simulink model "elevator"  (R2020a)
settings: Solver=VariableStepAuto  StartTime=0.0  StopTime=inf  RelTol=1e-3
PreLoadFcn:
  | slplc.api.loadDataTypes;
undefined symbols (not defined in the file): BOOL, DINT, INT, slplc
libraries: simulink x1
(part 34 of 38)

== matlab function elevator/PLCControllerSuite/__Logic/Task/Program/__Logic/OTE28/__Format ==
  data: BlockEnable input; RungIn input; RungOut input; data input
function setBlockFormat(BlockEnable, RungIn, RungOut, data)

if data~=0 && data~=1
    error('slplc:inivalidBooleanValue', 'Invalid boolean value %d', data);
end
data = logical(data);

% set parent block colors
coder.extrinsic('slplc.utils.setBlockAppearance');
persistent lastBlockEnable lastRungIn lastRungOut lastData isInit lastAnimation lastDataShow;
if isempty(lastBlockEnable)
    lastBlockEnable = true;
end
if isempty(lastRungIn)
    lastRungIn = false;
end
if isempty(lastRungOut)
    lastRungOut = false;
end
if isempty(lastData)
    lastData = data;
end
if isempty(isInit)
    isInit = true;
else
    isInit = false;
end
if isempty(lastAnimation)
    lastAnimation = false;
end
if isempty(lastDataShow)
    lastDataShow = false;
end

[animation, dataShow] = slplc.utils.setBlockAppearance('set', '%<PLCOperandTag>', {}, {}, ...
    ' = ', {'ForegroundColor'}, ...
    isInit,  ...
    BlockEnable, lastBlockEnable, ...
    RungIn,  lastRungIn, ...
    RungOut, lastRungOut, ...
    data, lastData, ...
    lastAnimation, lastDataShow);

lastBlockEnable = BlockEnable;
lastRungIn      = RungIn;
lastRungOut     = RungOut;
lastData        = data;
lastAnimation   = animation;
lastDataShow    = dataShow;
end

== matlab function elevator/PLCControllerSuite/__Logic/Task/Program/__Logic/XIC72/__Format ==
  data: BlockEnable input; RungIn input; RungOut input; data input
function setBlockFormat(BlockEnable, RungIn, RungOut, data)

if data~=0 && data~=1
    error('slplc:inivalidBooleanValue', 'Invalid boolean value %d', data);
end
data = logical(data);

% set parent block colors
coder.extrinsic('slplc.utils.setBlockAppearance');
persistent lastBlockEnable lastRungIn lastRungOut lastData isInit lastAnimation lastDataShow;
if isempty(lastBlockEnable)
    lastBlockEnable = true;
end
if isempty(lastRungIn)
    lastRungIn = false;
end
if isempty(lastRungOut)
    lastRungOut = false;
end
if isempty(lastData)
    lastData = data;
end
if isempty(isInit)
    isInit = true;
else
    isInit = false;
end
if isempty(lastAnimation)
    lastAnimation = false;
end
if isempty(lastDataShow)
    lastDataShow = false;
end

[animation, dataShow] = slplc.utils.setBlockAppearance('set', '%<PLCOperandTag>', {}, {}, ...
    ' = ', {'ForegroundColor'}, ...
    isInit,  ...
    BlockEnable, lastBlockEnable, ...
    RungIn,  lastRungIn, ...
    RungOut, lastRungOut, ...
    data, lastData, ...
    lastAnimation, lastDataShow);

lastBlockEnable = BlockEnable;
lastRungIn      = RungIn;
lastRungOut     = RungOut;
lastData        = data;
lastAnimation   = animation;
lastDataShow    = dataShow;
end

== matlab function elevator/PLCControllerSuite/__Logic/Task/Program/__Logic/XIO29/__Format ==
  data: BlockEnable input; RungIn input; RungOut input; data input
function setBlockFormat(BlockEnable, RungIn, RungOut, data)

if data~=0 && data~=1
    error('slplc:inivalidBooleanValue', 'Invalid boolean value %d', data);
end
data = logical(data);

% set parent block colors
coder.extrinsic('slplc.utils.setBlockAppearance');
persistent lastBlockEnable lastRungIn lastRungOut lastData isInit lastAnimation lastDataShow;
if isempty(lastBlockEnable)
    lastBlockEnable = true;
end
if isempty(lastRungIn)
    lastRungIn = false;
end
if isempty(lastRungOut)
    lastRungOut = false;
end
if isempty(lastData)
    lastData = data;
end
if isempty(isInit)
    isInit = true;
else
    isInit = false;
end
if isempty(lastAnimation)
    lastAnimation = false;
end
if isempty(lastDataShow)
    lastDataShow = false;
end

[animation, dataShow] = slplc.utils.setBlockAppearance('set', '%<PLCOperandTag>', {}, {}, ...
    ' = ', {'ForegroundColor'}, ...
    isInit,  ...
    BlockEnable, lastBlockEnable, ...
    RungIn,  lastRungIn, ...
    RungOut, lastRungOut, ...
    data, lastData, ...
    lastAnimation, lastDataShow);

lastBlockEnable = BlockEnable;
lastRungIn      = RungIn;
lastRungOut     = RungOut;
lastData        = data;
lastAnimation   = animation;
lastDataShow    = dataShow;
end

== matlab function elevator/PLCControllerSuite/__Logic/Task/Program/__Logic/XIC92/__Format ==
  data: BlockEnable input; RungIn input; RungOut input; data input
function setBlockFormat(BlockEnable, RungIn, RungOut, data)

if data~=0 && data~=1
    error('slplc:inivalidBooleanValue', 'Invalid boolean value %d', data);
end
data = logical(data);

% set parent block colors
coder.extrinsic('slplc.utils.setBlockAppearance');
persistent lastBlockEnable lastRungIn lastRungOut lastData isInit lastAnimation lastDataShow;
if isempty(lastBlockEnable)
    lastBlockEnable = true;
end
if isempty(lastRungIn)
    lastRungIn = false;
end
if isempty(lastRungOut)
    lastRungOut = false;
end
if isempty(lastData)
    lastData = data;
end
if isempty(isInit)
    isInit = true;
else
    isInit = false;
end
if isempty(lastAnimation)
    lastAnimation = false;
end
if isempty(lastDataShow)
    lastDataShow = false;
end

[animation, dataShow] = slplc.utils.setBlockAppearance('set', '%<PLCOperandTag>', {}, {}, ...
    ' = ', {'ForegroundColor'}, ...
    isInit,  ...
    BlockEnable, lastBlockEnable, ...
    RungIn,  lastRungIn, ...
    RungOut, lastRungOut, ...
    data, lastData, ...
    lastAnimation, lastDataShow);

lastBlockEnable = BlockEnable;
lastRungIn      = RungIn;
lastRungOut     = RungOut;
lastData        = data;
lastAnimation   = animation;
lastDataShow    = dataShow;
end

== matlab function elevator/PLCControllerSuite/__Logic/Task/Program/__Logic/Junction3/__Format ==
  data: BlockEnable input; RungOut input
function setBlockFormat(BlockEnable, RungOut)
% set parent block colors
coder.extrinsic('slplc.utils.setBlockAppearance');
persistent lastBlockEnable isInit lastRungOut lastAnimation lastRungOutShow;
if isempty(lastBlockEnable)
    lastBlockEnable = true;
end

if isempty(isInit)
    isInit = true;
else
    isInit = false;
end

if isempty(lastRungOut)
    lastRungOut = RungOut;
end

if isempty(lastAnimation)
    lastAnimation = false;
end

if isempty(lastRungOutShow)
    lastRungOutShow = false;
end

[animation, dataShow] = slplc.utils.setBlockAppearance('set', '', {'black', 'black'}, {}, ...
    '', {'ForegroundColor', 'BackgroundColor'}, ...
    isInit,  ...
    BlockEnable, lastBlockEnable, ...
    RungOut,   lastRungOut, ...
    RungOut,   lastRungOut, ...
    [],    [], ...
    lastAnimation, lastRungOutShow);

lastBlockEnable     = BlockEnable;
lastRungOut         = RungOut;
lastAnimation       = animation;
lastRungOutShow     = dataShow;
end

== matlab function elevator/PLCControllerSuite/__Logic/Task/Program/__Logic/XIC99/__Format ==
  data: BlockEnable input; RungIn input; RungOut input; data input
function setBlockFormat(BlockEnable, RungIn, RungOut, data)

if data~=0 && data~=1
    error('slplc:inivalidBooleanValue', 'Invalid boolean value %d', data);
end
data = logical(data);

% set parent block colors
coder.extrinsic('slplc.utils.setBlockAppearance');
persistent lastBlockEnable lastRungIn lastRungOut lastData isInit lastAnimation lastDataShow;
if isempty(lastBlockEnable)
    lastBlockEnable = true;
end
if isempty(lastRungIn)
    lastRungIn = false;
end
if isempty(lastRungOut)
    lastRungOut = false;
end
if isempty(lastData)
    lastData = data;
end
if isempty(isInit)
    isInit = true;
else
    isInit = false;
end
if isempty(lastAnimation)
    lastAnimation = false;
end
if isempty(lastDataShow)
    lastDataShow = false;
end

[animation, dataShow] = slplc.utils.setBlockAppearance('set', '%<PLCOperandTag>', {}, {}, ...
    ' = ', {'ForegroundColor'}, ...
    isInit,  ...
    BlockEnable, lastBlockEnable, ...
    RungIn,  lastRungIn, ...
    RungOut, lastRungOut, ...
    data, lastData, ...
    lastAnimation, lastDataShow);

lastBlockEnable = BlockEnable;
lastRungIn      = RungIn;
lastRungOut     = RungOut;
lastData        = data;
lastAnimation   = animation;
lastDataShow    = dataShow;
end

== matlab function elevator/PLCControllerSuite/__Logic/Task/Program/__Logic/XIO18/__Format ==
  data: BlockEnable input; RungIn input; RungOut input; data input
function setBlockFormat(BlockEnable, RungIn, RungOut, data)

if data~=0 && data~=1
    error('slplc:inivalidBooleanValue', 'Invalid boolean value %d', data);
end
data = logical(data);

% set parent block colors
coder.extrinsic('slplc.utils.setBlockAppearance');
persistent lastBlockEnable lastRungIn lastRungOut lastData isInit lastAnimation lastDataShow;
if isempty(lastBlockEnable)
    lastBlockEnable = true;
end
if isempty(lastRungIn)
    lastRungIn = false;
end
if isempty(lastRungOut)
    lastRungOut = false;
end
if isempty(lastData)
    lastData = data;
end
if isempty(isInit)
    isInit = true;
else
    isInit = false;
end
if isempty(lastAnimation)
    lastAnimation = false;
end
if isempty(lastDataShow)
    lastDataShow = false;
end

[animation, dataShow] = slplc.utils.setBlockAppearance('set', '%<PLCOperandTag>', {}, {}, ...
    ' = ', {'ForegroundColor'}, ...
    isInit,  ...
    BlockEnable, lastBlockEnable, ...
    RungIn,  lastRungIn, ...
    RungOut, lastRungOut, ...
    data, lastData, ...
    lastAnimation, lastDataShow);

lastBlockEnable = BlockEnable;
lastRungIn      = RungIn;
lastRungOut     = RungOut;
lastData        = data;
lastAnimation   = animation;
lastDataShow    = dataShow;
end

== matlab function elevator/PLCControllerSuite/__Logic/Task/Program/__Logic/XIO19/__Format ==
  data: BlockEnable input; RungIn input; RungOut input; data input
function setBlockFormat(BlockEnable, RungIn, RungOut, data)

if data~=0 && data~=1
    error('slplc:inivalidBooleanValue', 'Invalid boolean value %d', data);
end
data = logical(data);

% set parent block colors
coder.extrinsic('slplc.utils.setBlockAppearance');
persistent lastBlockEnable lastRungIn lastRungOut lastData isInit lastAnimation lastDataShow;
if isempty(lastBlockEnable)
    lastBlockEnable = true;
end
if isempty(lastRungIn)
    lastRungIn = false;
end
if isempty(lastRungOut)
    lastRungOut = false;
end
if isempty(lastData)
    lastData = data;
end
if isempty(isInit)
    isInit = true;
else
    isInit = false;
end
if isempty(lastAnimation)
    lastAnimation = false;
end
if isempty(lastDataShow)
    lastDataShow = false;
end

[animation, dataShow] = slplc.utils.setBlockAppearance('set', '%<PLCOperandTag>', {}, {}, ...
    ' = ', {'ForegroundColor'}, ...
    isInit,  ...
    BlockEnable, lastBlockEnable, ...
    RungIn,  lastRungIn, ...
    RungOut, lastRungOut, ...
    data, lastData, ...
    lastAnimation, lastDataShow);

lastBlockEnable = BlockEnable;
lastRungIn      = RungIn;
lastRungOut     = RungOut;
lastData        = data;
lastAnimation   = animation;
lastDataShow    = dataShow;
end

== matlab function elevator/PLCControllerSuite/__Logic/Task/Program/__Logic/XIO20/__Format ==
  data: BlockEnable input; RungIn input; RungOut input; data input
function setBlockFormat(BlockEnable, RungIn, RungOut, data)

if data~=0 && data~=1
    error('slplc:inivalidBooleanValue', 'Invalid boolean value %d', data);
end
data = logical(data);

% set parent block colors
coder.extrinsic('slplc.utils.setBlockAppearance');
persistent lastBlockEnable lastRungIn lastRungOut lastData isInit lastAnimation lastDataShow;
if isempty(lastBlockEnable)
    lastBlockEnable = true;
end
if isempty(lastRungIn)
    lastRungIn = false;
end
if isempty(lastRungOut)
    lastRungOut = false;
end
if isempty(lastData)
    lastData = data;
end
if isempty(isInit)
    isInit = true;
else
    isInit = false;
end
if isempty(lastAnimation)
    lastAnimation = false;
end
if isempty(lastDataShow)
    lastDataShow = false;
end

[animation, dataShow] = slplc.utils.setBlockAppearance('set', '%<PLCOperandTag>', {}, {}, ...
    ' = ', {'ForegroundColor'}, ...
    isInit,  ...
    BlockEnable, lastBlockEnable, ...
    RungIn,  lastRungIn, ...
    RungOut, lastRungOut, ...
    data, lastData, ...
    lastAnimation, lastDataShow);

lastBlockEnable = BlockEnable;
lastRungIn      = RungIn;
lastRungOut     = RungOut;
lastData        = data;
lastAnimation   = animation;
lastDataShow    = dataShow;
end

== matlab function elevator/PLCControllerSuite/__Logic/Task/Program/__Logic/XIO21/__Format ==
  data: BlockEnable input; RungIn input; RungOut input; data input
function setBlockFormat(BlockEnable, RungIn, RungOut, data)

if data~=0 && data~=1
    error('slplc:inivalidBooleanValue', 'Invalid boolean value %d', data);
end
data = logical(data);

% set parent block colors
coder.extrinsic('slplc.utils.setBlockAppearance');
persistent lastBlockEnable lastRungIn lastRungOut lastData isInit lastAnimation lastDataShow;
if isempty(lastBlockEnable)
    lastBlockEnable = true;
end
if isempty(lastRungIn)
    lastRungIn = false;
end
if isempty(lastRungOut)
    lastRungOut = false;
end
if isempty(lastData)
    lastData = data;
end
if isempty(isInit)
    isInit = true;
else
    isInit = false;
end
if isempty(lastAnimation)
    lastAnimation = false;
end
if isempty(lastDataShow)
    lastDataShow = false;
end

[animation, dataShow] = slplc.utils.setBlockAppearance('set', '%<PLCOperandTag>', {}, {}, ...
    ' = ', {'ForegroundColor'}, ...
    isInit,  ...
    BlockEnable, lastBlockEnable, ...
    RungIn,  lastRungIn, ...
    RungOut, lastRungOut, ...
    data, lastData, ...
    lastAnimation, lastDataShow);

lastBlockEnable = BlockEnable;
lastRungIn      = RungIn;
lastRungOut     = RungOut;
lastData        = data;
lastAnimation   = animation;
lastDataShow    = dataShow;
end

== matlab function elevator/PLCControllerSuite/__Logic/Task/Program/__Logic/XIO22/__Format ==
  data: BlockEnable input; RungIn input; RungOut input; data input
function setBlockFormat(BlockEnable, RungIn, RungOut, data)

if data~=0 && data~=1
    error('slplc:inivalidBooleanValue', 'Invalid boolean value %d', data);
end
data = logical(data);

% set parent block colors
coder.extrinsic('slplc.utils.setBlockAppearance');
persistent lastBlockEnable lastRungIn lastRungOut lastData isInit lastAnimation lastDataShow;
if isempty(lastBlockEnable)
    lastBlockEnable = true;
end
if isempty(lastRungIn)
    lastRungIn = false;
end
if isempty(lastRungOut)
    lastRungOut = false;
end
if isempty(lastData)
    lastData = data;
end
if isempty(isInit)
    isInit = true;
else
    isInit = false;
end
if isempty(lastAnimation)
    lastAnimation = false;
end
if isempty(lastDataShow)
    lastDataShow = false;
end

[animation, dataShow] = slplc.utils.setBlockAppearance('set', '%<PLCOperandTag>', {}, {}, ...
    ' = ', {'ForegroundColor'}, ...
    isInit,  ...
    BlockEnable, lastBlockEnable, ...
    RungIn,  lastRungIn, ...
    RungOut, lastRungOut, ...
    data, lastData, ...
    lastAnimation, lastDataShow);

lastBlockEnable = BlockEnable;
lastRungIn      = RungIn;
lastRungOut     = RungOut;
lastData        = data;
lastAnimation   = animation;
lastDataShow    = dataShow;
end

== matlab function elevator/PLCControllerSuite/__Logic/Task/Program/__Logic/XIO34/__Format ==
  data: BlockEnable input; RungIn input; RungOut input; data input
function setBlockFormat(BlockEnable, RungIn, RungOut, data)

if data~=0 && data~=1
    error('slplc:inivalidBooleanValue', 'Invalid boolean value %d', data);
end
data = logical(data);

% set parent block colors
coder.extrinsic('slplc.utils.setBlockAppearance');
persistent lastBlockEnable lastRungIn lastRungOut lastData isInit lastAnimation lastDataShow;
if isempty(lastBlockEnable)
    lastBlockEnable = true;
end
if isempty(lastRungIn)
    lastRungIn = false;
end
if isempty(lastRungOut)
    lastRungOut = false;
end
if isempty(lastData)
    lastData = data;
end
if isempty(isInit)
    isInit = true;
else
    isInit = false;
end
if isempty(lastAnimation)
    lastAnimation = false;
end
if isempty(lastDataShow)
    lastDataShow = false;
end

[animation, dataShow] = slplc.utils.setBlockAppearance('set', '%<PLCOperandTag>', {}, {}, ...
    ' = ', {'ForegroundColor'}, ...
    isInit,  ...
    BlockEnable, lastBlockEnable, ...
    RungIn,  lastRungIn, ...
    RungOut, lastRungOut, ...
    data, lastData, ...
    lastAnimation, lastDataShow);

lastBlockEnable = BlockEnable;
lastRungIn      = RungIn;
lastRungOut     = RungOut;
lastData        = data;
lastAnimation   = animation;
lastDataShow    = dataShow;
end

== matlab function elevator/PLCControllerSuite/__Logic/Task/Program/__Logic/Junction28/__Format ==
  data: BlockEnable input; RungOut input
function setBlockFormat(BlockEnable, RungOut)
% set parent block colors
coder.extrinsic('slplc.utils.setBlockAppearance');
persistent lastBlockEnable isInit lastRungOut lastAnimation lastRungOutShow;
if isempty(lastBlockEnable)
    lastBlockEnable = true;
end

if isempty(isInit)
    isInit = true;
else
    isInit = false;
end

if isempty(lastRungOut)
    lastRungOut = RungOut;
end

if isempty(lastAnimation)
    lastAnimation = false;
end

if isempty(lastRungOutShow)
    lastRungOutShow = false;
end

[animation, dataShow] = slplc.utils.setBlockAppearance('set', '', {'black', 'black'}, {}, ...
    '', {'ForegroundColor', 'BackgroundColor'}, ...
    isInit,  ...
    BlockEnable, lastBlockEnable, ...
    RungOut,   lastRungOut, ...
    RungOut,   lastRungOut, ...
    [],    [], ...
    lastAnimation, lastRungOutShow);

lastBlockEnable     = BlockEnable;
lastRungOut         = RungOut;
lastAnimation       = animation;
lastRungOutShow     = dataShow;
end

== matlab function elevator/PLCControllerSuite/__Logic/Task/Program/__Logic/OTE3/__Format ==
  data: BlockEnable input; RungIn input; RungOut input; data input
function setBlockFormat(BlockEnable, RungIn, RungOut, data)

if data~=0 && data~=1
    error('slplc:inivalidBooleanValue', 'Invalid boolean value %d', data);
end
data = logical(data);

% set parent block colors
coder.extrinsic('slplc.utils.setBlockAppearance');
persistent lastBlockEnable lastRungIn lastRungOut lastData isInit lastAnimation lastDataShow;
if isempty(lastBlockEnable)
    lastBlockEnable = true;
end
if isempty(lastRungIn)
    lastRungIn = false;
end
if isempty(lastRungOut)
    lastRungOut = false;
end
if isempty(lastData)
    lastData = data;
end
if isempty(isInit)
    isInit = true;
else
    isInit = false;
end
if isempty(lastAnimation)
    lastAnimation = false;
end
if isempty(lastDataShow)
    lastDataShow = false;
end

[animation, dataShow] = slplc.utils.setBlockAppearance('set', '%<PLCOperandTag>', {}, {}, ...
    ' = ', {'ForegroundColor'}, ...
    isInit,  ...
    BlockEnable, lastBlockEnable, ...
    RungIn,  lastRungIn, ...
    RungOut, lastRungOut, ...
    data, lastData, ...
    lastAnimation, lastDataShow);

lastBlockEnable = BlockEnable;
lastRungIn      = RungIn;
lastRungOut     = RungOut;
lastData        = data;
lastAnimation   = animation;
lastDataShow    = dataShow;
end

== matlab function elevator/PLCControllerSuite/__Logic/Task/Program/__Logic/OTE16/__Format ==
  data: BlockEnable input; RungIn input; RungOut input; data input
function setBlockFormat(BlockEnable, RungIn, RungOut, data)

if data~=0 && data~=1
    error('slplc:inivalidBooleanValue', 'Invalid boolean value %d', data);
end
data = logical(data);

% set parent block colors
coder.extrinsic('slplc.utils.setBlockAppearance');
persistent lastBlockEnable lastRungIn lastRungOut lastData isInit lastAnimation lastDataShow;
if isempty(lastBlockEnable)
    lastBlockEnable = true;
end
if isempty(lastRungIn)
    lastRungIn = false;
end
if isempty(lastRungOut)
    lastRungOut = false;
end
if isempty(lastData)
    lastData = data;
end
if isempty(isInit)
    isInit = true;
else
    isInit = false;
end
if isempty(lastAnimation)
    lastAnimation = false;
end
if isempty(lastDataShow)
    lastDataShow = false;
end

[animation, dataShow] = slplc.utils.setBlockAppearance('set', '%<PLCOperandTag>', {}, {}, ...
    ' = ', {'ForegroundColor'}, ...
    isInit,  ...
    BlockEnable, lastBlockEnable, ...
    RungIn,  lastRungIn, ...
    RungOut, lastRungOut, ...
    data, lastData, ...
    lastAnimation, lastDataShow);

lastBlockEnable = BlockEnable;
lastRungIn      = RungIn;
lastRungOut     = RungOut;
lastData        = data;
lastAnimation   = animation;
lastDataShow    = dataShow;
end

== matlab function elevator/PLCControllerSuite/__Logic/Task/Program/__Logic/XIC90/__Format ==
  data: BlockEnable input; RungIn input; RungOut input; data input
function setBlockFormat(BlockEnable, RungIn, RungOut, data)

if data~=0 && data~=1
    error('slplc:inivalidBooleanValue', 'Invalid boolean value %d', data);
end
data = logical(data);

% set parent block colors
coder.extrinsic('slplc.utils.setBlockAppearance');
persistent lastBlockEnable lastRungIn lastRungOut lastData isInit lastAnimation lastDataShow;
if isempty(lastBlockEnable)
    lastBlockEnable = true;
end
if isempty(lastRungIn)
    lastRungIn = false;
end
if isempty(lastRungOut)
    lastRungOut = false;
end
if isempty(lastData)
    lastData = data;
end
if isempty(isInit)
    isInit = true;
else
    isInit = false;
end
if isempty(lastAnimation)
    lastAnimation = false;
end
if isempty(lastDataShow)
    lastDataShow = false;
end

[animation, dataShow] = slplc.utils.setBlockAppearance('set', '%<PLCOperandTag>', {}, {}, ...
    ' = ', {'ForegroundColor'}, ...
    isInit,  ...
    BlockEnable, lastBlockEnable, ...
    RungIn,  lastRungIn, ...
    RungOut, lastRungOut, ...
    data, lastData, ...
    lastAnimation, lastDataShow);

lastBlockEnable = BlockEnable;
lastRungIn      = RungIn;
lastRungOut     = RungOut;
lastData        = data;
lastAnimation   = animation;
lastDataShow    = dataShow;
end

== matlab function elevator/PLCControllerSuite/__Logic/Task/Program/__Logic/XIC91/__Format ==
  data: BlockEnable input; RungIn input; RungOut input; data input
function setBlockFormat(BlockEnable, RungIn, RungOut, data)

if data~=0 && data~=1
    error('slplc:inivalidBooleanValue', 'Invalid boolean value %d', data);
end
data = logical(data);

% set parent block colors
coder.extrinsic('slplc.utils.setBlockAppearance');
persistent lastBlockEnable lastRungIn lastRungOut lastData isInit lastAnimation lastDataShow;
if isempty(lastBlockEnable)
    lastBlockEnable = true;
end
if isempty(lastRungIn)
    lastRungIn = false;
end
if isempty(lastRungOut)
    lastRungOut = false;
end
if isempty(lastData)
    lastData = data;
end
if isempty(isInit)
    isInit = true;
else
    isInit = false;
end
if isempty(lastAnimation)
    lastAnimation = false;
end
if isempty(lastDataShow)
    lastDataShow = false;
end

[animation, dataShow] = slplc.utils.setBlockAppearance('set', '%<PLCOperandTag>', {}, {}, ...
    ' = ', {'ForegroundColor'}, ...
    isInit,  ...
    BlockEnable, lastBlockEnable, ...
    RungIn,  lastRungIn, ...
    RungOut, lastRungOut, ...
    data, lastData, ...
    lastAnimation, lastDataShow);

lastBlockEnable = BlockEnable;
lastRungIn      = RungIn;
lastRungOut     = RungOut;
lastData        = data;
lastAnimation   = animation;
lastDataShow    = dataShow;
end

== matlab function elevator/PLCControllerSuite/__Logic/Task/Program/__Logic/Junction32/__Format ==
  data: BlockEnable input; RungOut input
function setBlockFormat(BlockEnable, RungOut)
% set parent block colors
coder.extrinsic('slplc.utils.setBlockAppearance');
persistent lastBlockEnable isInit lastRungOut lastAnimation lastRungOutShow;
if isempty(lastBlockEnable)
    lastBlockEnable = true;
end

if isempty(isInit)
    isInit = true;
else
    isInit = false;
end

if isempty(lastRungOut)
    lastRungOut = RungOut;
end

if isempty(lastAnimation)
    lastAnimation = false;
end

if isempty(lastRungOutShow)
    lastRungOutShow = false;
end

[animation, dataShow] = slplc.utils.setBlockAppearance('set', '', {'black', 'black'}, {}, ...
    '', {'ForegroundColor', 'BackgroundColor'}, ...
    isInit,  ...
    BlockEnable, lastBlockEnable, ...
    RungOut,   lastRungOut, ...
    RungOut,   lastRungOut, ...
    [],    [], ...
    lastAnimation, lastRungOutShow);

lastBlockEnable     = BlockEnable;
lastRungOut         = RungOut;
lastAnimation       = animation;
lastRungOutShow     = dataShow;
end

== matlab function elevator/PLCControllerSuite/__Logic/Task/Program/__Logic/OTE21/__Format ==
  data: BlockEnable input; RungIn input; RungOut input; data input
function setBlockFormat(BlockEnable, RungIn, RungOut, data)

if data~=0 && data~=1
    error('slplc:inivalidBooleanValue', 'Invalid boolean value %d', data);
end
data = logical(data);

% set parent block colors
coder.extrinsic('slplc.utils.setBlockAppearance');
persistent lastBlockEnable lastRungIn lastRungOut lastData isInit lastAnimation lastDataShow;
if isempty(lastBlockEnable)
    lastBlockEnable = true;
end
if isempty(lastRungIn)
    lastRungIn = false;
end
if isempty(lastRungOut)
    lastRungOut = false;
end
if isempty(lastData)
    lastData = data;
end
if isempty(isInit)
    isInit = true;
else
    isInit = false;
end
if isempty(lastAnimation)
    lastAnimation = false;
end
if isempty(lastDataShow)
    lastDataShow = false;
end

[animation, dataShow] = slplc.utils.setBlockAppearance('set', '%<PLCOperandTag>', {}, {}, ...
    ' = ', {'ForegroundColor'}, ...
    isInit,  ...
    BlockEnable, lastBlockEnable, ...
    RungIn,  lastRungIn, ...
    RungOut, lastRungOut, ...
    data, lastData, ...
    lastAnimation, lastDataShow);

lastBlockEnable = BlockEnable;
lastRungIn      = RungIn;
lastRungOut     = RungOut;
lastData        = data;
lastAnimation   = animation;
lastDataShow    = dataShow;
end

== matlab function elevator/PLCControllerSuite/__Logic/Task/Program/__Logic/XIC93/__Format ==
  data: BlockEnable input; RungIn input; RungOut input; data input
function setBlockFormat(BlockEnable, RungIn, RungOut, data)

if data~=0 && data~=1
    error('slplc:inivalidBooleanValue', 'Invalid boolean value %d', data);
end
data = logical(data);

% set parent block colors
coder.extrinsic('slplc.utils.setBlockAppearance');
persistent lastBlockEnable lastRungIn lastRungOut lastData isInit lastAnimation lastDataShow;
if isempty(lastBlockEnable)
    lastBlockEnable = true;
end
if isempty(lastRungIn)
    lastRungIn = false;
end
if isempty(lastRungOut)
    lastRungOut = false;
end
if isempty(lastData)
    lastData = data;
end
if isempty(isInit)
    isInit = true;
else
    isInit = false;
end
if isempty(lastAnimation)
    lastAnimation = false;
end
if isempty(lastDataShow)
    lastDataShow = false;
end

[animation, dataShow] = slplc.utils.setBlockAppearance('set', '%<PLCOperandTag>', {}, {}, ...
    ' = ', {'ForegroundColor'}, ...
    isInit,  ...
    BlockEnable, lastBlockEnable, ...
    RungIn,  lastRungIn, ...
    RungOut, lastRungOut, ...
    data, lastData, ...
    lastAnimation, lastDataShow);

lastBlockEnable = BlockEnable;
lastRungIn      = RungIn;
lastRungOut     = RungOut;
lastData        = data;
lastAnimation   = animation;
lastDataShow    = dataShow;
end

== matlab function elevator/PLCControllerSuite/__Logic/Task/Program/__Logic/XIC94/__Format ==
  data: BlockEnable input; RungIn input; RungOut input; data input
function setBlockFormat(BlockEnable, RungIn, RungOut, data)

if data~=0 && data~=1
    error('slplc:inivalidBooleanValue', 'Invalid boolean value %d', data);
end
data = logical(data);

% set parent block colors
coder.extrinsic('slplc.utils.setBlockAppearance');
persistent lastBlockEnable lastRungIn lastRungOut lastData isInit lastAnimation lastDataShow;
if isempty(lastBlockEnable)
    lastBlockEnable = true;
end
if isempty(lastRungIn)
    lastRungIn = false;
end
if isempty(lastRungOut)
    lastRungOut = false;
end
if isempty(lastData)
    lastData = data;
end
if isempty(isInit)
    isInit = true;
else
    isInit = false;
end
if isempty(lastAnimation)
    lastAnimation = false;
end
if isempty(lastDataShow)
    lastDataShow = false;
end

[animation, dataShow] = slplc.utils.setBlockAppearance('set', '%<PLCOperandTag>', {}, {}, ...
    ' = ', {'ForegroundColor'}, ...
    isInit,  ...
    BlockEnable, lastBlockEnable, ...
    RungIn,  lastRungIn, ...
    RungOut, lastRungOut, ...
    data, lastData, ...
    lastAnimation, lastDataShow);

lastBlockEnable = BlockEnable;
lastRungIn      = RungIn;
lastRungOut     = RungOut;
lastData        = data;
lastAnimation   = animation;
lastDataShow    = dataShow;
end

== matlab function elevator/PLCControllerSuite/__Logic/Task/Program/__Logic/Junction33/__Format ==
  data: BlockEnable input; RungOut input
function setBlockFormat(BlockEnable, RungOut)
% set parent block colors
coder.extrinsic('slplc.utils.setBlockAppearance');
persistent lastBlockEnable isInit lastRungOut lastAnimation lastRungOutShow;
if isempty(lastBlockEnable)
    lastBlockEnable = true;
end

if isempty(isInit)
    isInit = true;
else
    isInit = false;
end

if isempty(lastRungOut)
    lastRungOut = RungOut;
end

if isempty(lastAnimation)
    lastAnimation = false;
end

if isempty(lastRungOutShow)
    lastRungOutShow = false;
end

[animation, dataShow] = slplc.utils.setBlockAppearance('set', '', {'black', 'black'}, {}, ...
    '', {'ForegroundColor', 'BackgroundColor'}, ...
    isInit,  ...
    BlockEnable, lastBlockEnable, ...
    RungOut,   lastRungOut, ...
    RungOut,   lastRungOut, ...
    [],    [], ...
    lastAnimation, lastRungOutShow);

lastBlockEnable     = BlockEnable;
lastRungOut         = RungOut;
lastAnimation       = animation;
lastRungOutShow     = dataShow;
end

== matlab function elevator/PLCControllerSuite/__Logic/Task/Program/__Logic/OTE22/__Format ==
  data: BlockEnable input; RungIn input; RungOut input; data input
function setBlockFormat(BlockEnable, RungIn, RungOut, data)

if data~=0 && data~=1
    error('slplc:inivalidBooleanValue', 'Invalid boolean value %d', data);
end
data = logical(data);

% set parent block colors
coder.extrinsic('slplc.utils.setBlockAppearance');
persistent lastBlockEnable lastRungIn lastRungOut lastData isInit lastAnimation lastDataShow;
if isempty(lastBlockEnable)
    lastBlockEnable = true;
end
if isempty(lastRungIn)
    lastRungIn = false;
end
if isempty(lastRungOut)
    lastRungOut = false;
end
if isempty(lastData)
    lastData = data;
end
if isempty(isInit)
    isInit = true;
else
    isInit = false;
end
if isempty(lastAnimation)
    lastAnimation = false;
end
if isempty(lastDataShow)
    lastDataShow = false;
end

[animation, dataShow] = slplc.utils.setBlockAppearance('set', '%<PLCOperandTag>', {}, {}, ...
    ' = ', {'ForegroundColor'}, ...
    isInit,  ...
    BlockEnable, lastBlockEnable, ...
    RungIn,  lastRungIn, ...
    RungOut, lastRungOut, ...
    data, lastData, ...
    lastAnimation, lastDataShow);

lastBlockEnable = BlockEnable;
lastRungIn      = RungIn;
lastRungOut     = RungOut;
lastData        = data;
lastAnimation   = animation;
lastDataShow    = dataShow;
end

== matlab function elevator/PLCControllerSuite/__Logic/Task/Program/__Logic/XIC95/__Format ==
  data: BlockEnable input; RungIn input; RungOut input; data input
function setBlockFormat(BlockEnable, RungIn, RungOut, data)

if data~=0 && data~=1
    error('slplc:inivalidBooleanValue', 'Invalid boolean value %d', data);
end
data = logical(data);

% set parent block colors
coder.extrinsic('slplc.utils.setBlockAppearance');
persistent lastBlockEnable lastRungIn lastRungOut lastData isInit lastAnimation lastDataShow;
if isempty(lastBlockEnable)
    lastBlockEnable = true;
end
if isempty(lastRungIn)
    lastRungIn = false;
end
if isempty(lastRungOut)
    lastRungOut = false;
end
if isempty(lastData)
    lastData = data;
end
if isempty(isInit)
    isInit = true;
else
    isInit = false;
end
if isempty(lastAnimation)
    lastAnimation = false;
end
if isempty(lastDataShow)
    lastDataShow = false;
end

[animation, dataShow] = slplc.utils.setBlockAppearance('set', '%<PLCOperandTag>', {}, {}, ...
    ' = ', {'ForegroundColor'}, ...
    isInit,  ...
    BlockEnable, lastBlockEnable, ...
    RungIn,  lastRungIn, ...
    RungOut, lastRungOut, ...
    data, lastData, ...
    lastAnimation, lastDataShow);

lastBlockEnable = BlockEnable;
lastRungIn      = RungIn;
lastRungOut     = RungOut;
lastData        = data;
lastAnimation   = animation;
lastDataShow    = dataShow;
end

== matlab function elevator/PLCControllerSuite/__Logic/Task/Program/__Logic/XIC96/__Format ==
  data: BlockEnable input; RungIn input; RungOut input; data input
function setBlockFormat(BlockEnable, RungIn, RungOut, data)

if data~=0 && data~=1
    error('slplc:inivalidBooleanValue', 'Invalid boolean value %d', data);
end
data = logical(data);

% set parent block colors
coder.extrinsic('slplc.utils.setBlockAppearance');
persistent lastBlockEnable lastRungIn lastRungOut lastData isInit lastAnimation lastDataShow;
if isempty(lastBlockEnable)
    lastBlockEnable = true;
end
if isempty(lastRungIn)
    lastRungIn = false;
end
if isempty(lastRungOut)
    lastRungOut = false;
end
if isempty(lastData)
    lastData = data;
end
if isempty(isInit)
    isInit = true;
else
    isInit = false;
end
if isempty(lastAnimation)
    lastAnimation = false;
end
if isempty(lastDataShow)
    lastDataShow = false;
end

[animation, dataShow] = slplc.utils.setBlockAppearance('set', '%<PLCOperandTag>', {}, {}, ...
    ' = ', {'ForegroundColor'}, ...
    isInit,  ...
    BlockEnable, lastBlockEnable, ...
    RungIn,  lastRungIn, ...
    RungOut, lastRungOut, ...
    data, lastData, ...
    lastAnimation, lastDataShow);

lastBlockEnable = BlockEnable;
lastRungIn      = RungIn;
lastRungOut     = RungOut;
lastData        = data;
lastAnimation   = animation;
lastDataShow    = dataShow;
end

== matlab function elevator/PLCControllerSuite/__Logic/Task/Program/__Logic/XIC10/__Format ==
  data: BlockEnable input; RungIn input; RungOut input; data input
function setBlockFormat(BlockEnable, RungIn, RungOut, data)

if data~=0 && data~=1
    error('slplc:inivalidBooleanValue', 'Invalid boolean value %d', data);
end
data = logical(data);

% set parent block colors
coder.extrinsic('slplc.utils.setBlockAppearance');
persistent lastBlockEnable lastRungIn lastRungOut lastData isInit lastAnimation lastDataShow;
if isempty(lastBlockEnable)
    lastBlockEnable = true;
end
if isempty(lastRungIn)
    lastRungIn = false;
end
if isempty(lastRungOut)
    lastRungOut = false;
end
if isempty(lastData)
    lastData = data;
end
if isempty(isInit)
    isInit = true;
else
    isInit = false;
end
if isempty(lastAnimation)
    lastAnimation = false;
end
if isempty(lastDataShow)
    lastDataShow = false;
end

[animation, dataShow] = slplc.utils.setBlockAppearance('set', '%<PLCOperandTag>', {}, {}, ...
    ' = ', {'ForegroundColor'}, ...
    isInit,  ...
    BlockEnable, lastBlockEnable, ...
    RungIn,  lastRungIn, ...
    RungOut, lastRungOut, ...
    data, lastData, ...
    lastAnimation, lastDataShow);

lastBlockEnable = BlockEnable;
lastRungIn      = RungIn;
lastRungOut     = RungOut;
lastData        = data;
lastAnimation   = animation;
lastDataShow    = dataShow;
end

== matlab function elevator/PLCControllerSuite/__Logic/Task/Program/__Logic/Junction29/__Format ==
  data: BlockEnable input; RungOut input
function setBlockFormat(BlockEnable, RungOut)
% set parent block colors
coder.extrinsic('slplc.utils.setBlockAppearance');
persistent lastBlockEnable isInit lastRungOut lastAnimation lastRungOutShow;
if isempty(lastBlockEnable)
    lastBlockEnable = true;
end

if isempty(isInit)
    isInit = true;
else
    isInit = false;
end

if isempty(lastRungOut)
    lastRungOut = RungOut;
end

if isempty(lastAnimation)
    lastAnimation = false;
end

if isempty(lastRungOutShow)
    lastRungOutShow = false;
end

[animation, dataShow] = slplc.utils.setBlockAppearance('set', '', {'black', 'black'}, {}, ...
    '', {'ForegroundColor', 'BackgroundColor'}, ...
    isInit,  ...
    BlockEnable, lastBlockEnable, ...
    RungOut,   lastRungOut, ...
    RungOut,   lastRungOut, ...
    [],    [], ...
    lastAnimation, lastRungOutShow);

lastBlockEnable     = BlockEnable;
lastRungOut         = RungOut;
lastAnimation       = animation;
lastRungOutShow     = dataShow;
end

== matlab function elevator/PLCControllerSuite/__Logic/Task/Program/__Logic/XIC40/__Format ==
  data: BlockEnable input; RungIn input; RungOut input; data input
function setBlockFormat(BlockEnable, RungIn, RungOut, data)

if data~=0 && data~=1
    error('slplc:inivalidBooleanValue', 'Invalid boolean value %d', data);
end
data = logical(data);

% set parent block colors
coder.extrinsic('slplc.utils.setBlockAppearance');
persistent lastBlockEnable lastRungIn lastRungOut lastData isInit lastAnimation lastDataShow;
if isempty(lastBlockEnable)
    lastBlockEnable = true;
end
if isempty(lastRungIn)
    lastRungIn = false;
end
if isempty(lastRungOut)
    lastRungOut = false;
end
if isempty(lastData)
    lastData = data;
end
if isempty(isInit)
    isInit = true;
else
    isInit = false;
end
if isempty(lastAnimation)
    lastAnimation = false;
end
if isempty(lastDataShow)
    lastDataShow = false;
end

[animation, dataShow] = slplc.utils.setBlockAppearance('set', '%<PLCOperandTag>', {}, {}, ...
    ' = ', {'ForegroundColor'}, ...
    isInit,  ...
    BlockEnable, lastBlockEnable, ...
    RungIn,  lastRungIn, ...
    RungOut, lastRungOut, ...
    data, lastData, ...
    lastAnimation, lastDataShow);

lastBlockEnable = BlockEnable;
lastRungIn      = RungIn;
lastRungOut     = RungOut;
lastData        = data;
lastAnimation   = animation;
lastDataShow    = dataShow;
end

== matlab function elevator/PLCControllerSuite/__Logic/Task/Program/__Logic/Junction34/__Format ==
  data: BlockEnable input; RungOut input
function setBlockFormat(BlockEnable, RungOut)
% set parent block colors
coder.extrinsic('slplc.utils.setBlockAppearance');
persistent lastBlockEnable isInit lastRungOut lastAnimation lastRungOutShow;
if isempty(lastBlockEnable)
    lastBlockEnable = true;
end

if isempty(isInit)
    isInit = true;
else
    isInit = false;
end

if isempty(lastRungOut)
    lastRungOut = RungOut;
end

if isempty(lastAnimation)
    lastAnimation = false;
end

if isempty(lastRungOutShow)
    lastRungOutShow = false;
end

[animation, dataShow] = slplc.utils.setBlockAppearance('set', '', {'black', 'black'}, {}, ...
    '', {'ForegroundColor', 'BackgroundColor'}, ...
    isInit,  ...
    BlockEnable, lastBlockEnable, ...
    RungOut,   lastRungOut, ...
    RungOut,   lastRungOut, ...
    [],    [], ...
    lastAnimation, lastRungOutShow);

lastBlockEnable     = BlockEnable;
lastRungOut         = RungOut;
lastAnimation       = animation;
lastRungOutShow     = dataShow;
end

== matlab function elevator/PLCControllerSuite/__Logic/Task/Program/__Logic/XIO30/__Format ==
  data: BlockEnable input; RungIn input; RungOut input; data input
function setBlockFormat(BlockEnable, RungIn, RungOut, data)

if data~=0 && data~=1
    error('slplc:inivalidBooleanValue', 'Invalid boolean value %d', data);
end
data = logical(data);

% set parent block colors
coder.extrinsic('slplc.utils.setBlockAppearance');
persistent lastBlockEnable lastRungIn lastRungOut lastData isInit lastAnimation lastDataShow;
if isempty(lastBlockEnable)
    lastBlockEnable = true;
end
if isempty(lastRungIn)
    lastRungIn = false;
end
if isempty(lastRungOut)
    lastRungOut = false;
end
if isempty(lastData)
    lastData = data;
end
if isempty(isInit)
    isInit = true;
else
    isInit = false;
end
if isempty(lastAnimation)
    lastAnimation = false;
end
if isempty(lastDataShow)
    lastDataShow = false;
end

[animation, dataShow] = slplc.utils.setBlockAppearance('set', '%<PLCOperandTag>', {}, {}, ...
    ' = ', {'ForegroundColor'}, ...
    isInit,  ...
    BlockEnable, lastBlockEnable, ...
    RungIn,  lastRungIn, ...
    RungOut, lastRungOut, ...
    data, lastData, ...
    lastAnimation, lastDataShow);

lastBlockEnable = BlockEnable;
lastRungIn      = RungIn;
lastRungOut     = RungOut;
lastData        = data;
lastAnimation   = animation;
lastDataShow    = dataShow;
end

== matlab function elevator/PLCControllerSuite/__Logic/Task/Program/__Logic/OTE12/__Format ==
  data: BlockEnable input; RungIn input; RungOut input; data input
function setBlockFormat(BlockEnable, RungIn, RungOut, data)

if data~=0 && data~=1
    error('slplc:inivalidBooleanValue', 'Invalid boolean value %d', data);
end
data = logical(data);

% set parent block colors
coder.extrinsic('slplc.utils.setBlockAppearance');
persistent lastBlockEnable lastRungIn lastRungOut lastData isInit lastAnimation lastDataShow;
if isempty(lastBlockEnable)
    lastBlockEnable = true;
end
if isempty(lastRungIn)
    lastRungIn = false;
end
if isempty(lastRungOut)
    lastRungOut = false;
end
if isempty(lastData)
    lastData = data;
end
if isempty(isInit)
    isInit = true;
else
    isInit = false;
end
if isempty(lastAnimation)
    lastAnimation = false;
end
if isempty(lastDataShow)
    lastDataShow = false;
end

[animation, dataShow] = slplc.utils.setBlockAppearance('set', '%<PLCOperandTag>', {}, {}, ...
    ' = ', {'ForegroundColor'}, ...
    isInit,  ...
    BlockEnable, lastBlockEnable, ...
    RungIn,  lastRungIn, ...
    RungOut, lastRungOut, ...
    data, lastData, ...
    lastAnimation, lastDataShow);

lastBlockEnable = BlockEnable;
lastRungIn      = RungIn;
lastRungOut     = RungOut;
lastData        = data;
lastAnimation   = animation;
lastDataShow    = dataShow;
end

== matlab function elevator/PLCControllerSuite/__Logic/Task/Program/__Logic/OTE14/__Format ==
  data: BlockEnable input; RungIn input; RungOut input; data input
function setBlockFormat(BlockEnable, RungIn, RungOut, data)

if data~=0 && data~=1
    error('slplc:inivalidBooleanValue', 'Invalid boolean value %d', data);
end
data = logical(data);

% set parent block colors
coder.extrinsic('slplc.utils.setBlockAppearance');
persistent lastBlockEnable lastRungIn lastRungOut lastData isInit lastAnimation lastDataShow;
if isempty(lastBlockEnable)
    lastBlockEnable = true;
end
if isempty(lastRungIn)
    lastRungIn = false;
end
if isempty(lastRungOut)
    lastRungOut = false;
end
if isempty(lastData)
    lastData = data;
end
if isempty(isInit)
    isInit = true;
else
    isInit = false;
end
if isempty(lastAnimation)
    lastAnimation = false;
end
if isempty(lastDataShow)
    lastDataShow = false;
end

[animation, dataShow] = slplc.utils.setBlockAppearance('set', '%<PLCOperandTag>', {}, {}, ...
    ' = ', {'ForegroundColor'}, ...
    isInit,  ...
    BlockEnable, lastBlockEnable, ...
    RungIn,  lastRungIn, ...
    RungOut, lastRungOut, ...
    data, lastData, ...
    lastAnimation, lastDataShow);

lastBlockEnable = BlockEnable;
lastRungIn      = RungIn;
lastRungOut     = RungOut;
lastData        = data;
lastAnimation   = animation;
lastDataShow    = dataShow;
end

== matlab function elevator/PLCControllerSuite/__Logic/Task/Program/__Logic/OTE29/__Format ==
  data: BlockEnable input; RungIn input; RungOut input; data input
function setBlockFormat(BlockEnable, RungIn, RungOut, data)

if data~=0 && data~=1
    error('slplc:inivalidBooleanValue', 'Invalid boolean value %d', data);
end
data = logical(data);

% set parent block colors
coder.extrinsic('slplc.utils.setBlockAppearance');
persistent lastBlockEnable lastRungIn lastRungOut lastData isInit lastAnimation lastDataShow;
if isempty(lastBlockEnable)
    lastBlockEnable = true;
end
if isempty(lastRungIn)
    lastRungIn = false;
end
if isempty(lastRungOut)
    lastRungOut = false;
end
if isempty(lastData)
    lastData = data;
end
if isempty(isInit)
    isInit = true;
else
    isInit = false;
end
if isempty(lastAnimation)
    lastAnimation = false;
end
if isempty(lastDataShow)
    lastDataShow = false;
end

[animation, dataShow] = slplc.utils.setBlockAppearance('set', '%<PLCOperandTag>', {}, {}, ...
    ' = ', {'ForegroundColor'}, ...
    isInit,  ...
    BlockEnable, lastBlockEnable, ...
    RungIn,  lastRungIn, ...
    RungOut, lastRungOut, ...
    data, lastData, ...
    lastAnimation, lastDataShow);

lastBlockEnable = BlockEnable;
lastRungIn      = RungIn;
lastRungOut     = RungOut;
lastData        = data;
lastAnimation   = animation;
lastDataShow    = dataShow;
end

== matlab function elevator/PLCControllerSuite/__Logic/Task/Program/__Logic/ADD/__Format ==
  data: BlockEnable input; RungIn input; RungOut input
function setBlockFormat(BlockEnable, RungIn, RungOut)
% set parent block colors
coder.extrinsic('slplc.utils.setBlockAppearance');
persistent lastBlockEnable lastRungIn lastRungOut isInit lastAnimation lastDataShow;
if isempty(lastBlockEnable)
    lastBlockEnable = true;
end
if isempty(lastRungIn)
    lastRungIn = false;
end
if isempty(lastRungOut)
    lastRungOut = false;
end

if isempty(isInit)
    isInit = true;
else
    isInit = false;
end
if isempty(lastAnimation)
    lastAnimation = false;
end
if isempty(lastDataShow)
    lastDataShow = false;
end

[animation, dataShow] = slplc.utils.setBlockAppearance('set', '', {}, {}, ...
    ' = ',  {'ForegroundColor'}, ...
    isInit,  ...
    BlockEnable, lastBlockEnable, ...
    RungIn,  lastRungIn, ...
    RungOut, lastRungOut, ...
    [],    [], ...
    lastAnimation, lastDataShow);

lastBlockEnable = BlockEnable;
lastRungIn      = RungIn;
lastRungOut     = RungOut;
lastAnimation   = animation;
lastDataShow    = dataShow;
end

== matlab function elevator/PLCControllerSuite/__Logic/Task/Program/__Logic/Variable Read10/__Format ==
  data: data input
function setBlockFormat(data)
% set parent block colors
coder.extrinsic('slplc.utils.setBlockAppearance');
persistent isInit lastData  lastAnimation lastDataShow;

if isempty(isInit)
    isInit = true;
else
    isInit = false;
end

if isempty(lastData)
    lastData = data;
end

if isempty(lastAnimation)
    lastAnimation = false;
end

if isempty(lastDataShow)
    lastDataShow = false;
end

[animation, dataShow] = slplc.utils.setBlockAppearance('set', '', {}, {}, ...
    '%<PLCOperandTag> = ', {}, ...
    isInit,  ...
    true,  true, ...
    false, false, ...
    false, false, ...
    data,  lastData, ...
    lastAnimation, lastDataShow);

lastData        = data;
lastAnimation   = animation;
lastDataShow    = dataShow;
end

== matlab function elevator/PLCControllerSuite/__Logic/Task/Program/__Logic/XIC102/__Format ==
  data: BlockEnable input; RungIn input; RungOut input; data input
function setBlockFormat(BlockEnable, RungIn, RungOut, data)

if data~=0 && data~=1
    error('slplc:inivalidBooleanValue', 'Invalid boolean value %d', data);
end
data = logical(data);

% set parent block colors
coder.extrinsic('slplc.utils.setBlockAppearance');
persistent lastBlockEnable lastRungIn lastRungOut lastData isInit lastAnimation lastDataShow;
if isempty(lastBlockEnable)
    lastBlockEnable = true;
end
if isempty(lastRungIn)
    lastRungIn = false;
end
if isempty(lastRungOut)
    lastRungOut = false;
end
if isempty(lastData)
    lastData = data;
end
if isempty(isInit)
    isInit = true;
else
    isInit = false;
end
if isempty(lastAnimation)
    lastAnimation = false;
end
if isempty(lastDataShow)
    lastDataShow = false;
end

[animation, dataShow] = slplc.utils.setBlockAppearance('set', '%<PLCOperandTag>', {}, {}, ...
    ' = ', {'ForegroundColor'}, ...
    isInit,  ...
    BlockEnable, lastBlockEnable, ...
    RungIn,  lastRungIn, ...
    RungOut, lastRungOut, ...
    data, lastData, ...
    lastAnimation, lastDataShow);

lastBlockEnable = BlockEnable;
lastRungIn      = RungIn;
lastRungOut     = RungOut;
lastData        = data;
lastAnimation   = animation;
lastDataShow    = dataShow;
end

== matlab function elevator/PLCControllerSuite/__Logic/Task/Program/__Logic/XIC11/__Format ==
  data: BlockEnable input; RungIn input; RungOut input; data input
function setBlockFormat(BlockEnable, RungIn, RungOut, data)

if data~=0 && data~=1
    error('slplc:inivalidBooleanValue', 'Invalid boolean value %d', data);
end
data = logical(data);

% set parent block colors
coder.extrinsic('slplc.utils.setBlockAppearance');
persistent lastBlockEnable lastRungIn lastRungOut lastData isInit lastAnimation lastDataShow;
if isempty(lastBlockEnable)
    lastBlockEnable = true;
end
if isempty(lastRungIn)
    lastRungIn = false;
end
if isempty(lastRungOut)
    lastRungOut = false;
end
if isempty(lastData)
    lastData = data;
end
if isempty(isInit)
    isInit = true;
else
    isInit = false;
end
if isempty(lastAnimation)
    lastAnimation = false;
end
if isempty(lastDataShow)
    lastDataShow = false;
end

[animation, dataShow] = slplc.utils.setBlockAppearance('set', '%<PLCOperandTag>', {}, {}, ...
    ' = ', {'ForegroundColor'}, ...
    isInit,  ...
    BlockEnable, lastBlockEnable, ...
    RungIn,  lastRungIn, ...
    RungOut, lastRungOut, ...
    data, lastData, ...
    lastAnimation, lastDataShow);

lastBlockEnable = BlockEnable;
lastRungIn      = RungIn;
lastRungOut     = RungOut;
lastData        = data;
lastAnimation   = animation;
lastDataShow    = dataShow;
end
